simulink model "lb3"  (R2023b)
settings: Solver=ode15s  StartTime=0.0  StopTime=10.0  MaxStep=1e-5  RelTol=1e-3
values from neighbouring files (symbols this model uses):
  C = [0, 1, 0, 0]    [lw3_1.m]
  H = acker(A, B, p_reg)    [lw3_1.m]    (also in lw3_2.m = zeros(1,4))
  K = acker(A', C', poles_obs)'    [lw3_1.m]
  x0 = [1; 0; 0; 0]    [lw3_1.m]
  x00 = [0; 0; 0; 0]    [lw3_1.m]
undefined symbols (not defined in the file or in its folder): A, B, G
settings Model: Creator=kek  LastModifiedBy=kek

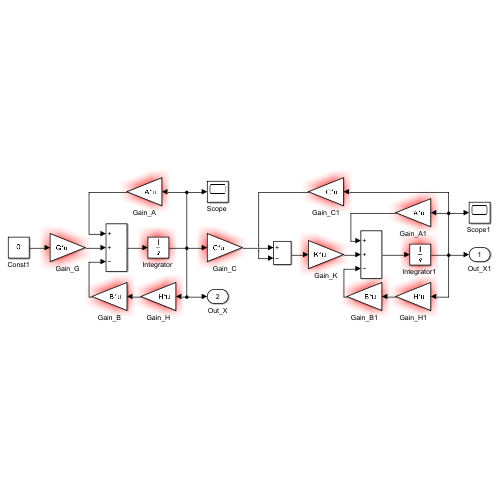
[thumbnail: Simulink's stored preview of the top-level diagram]
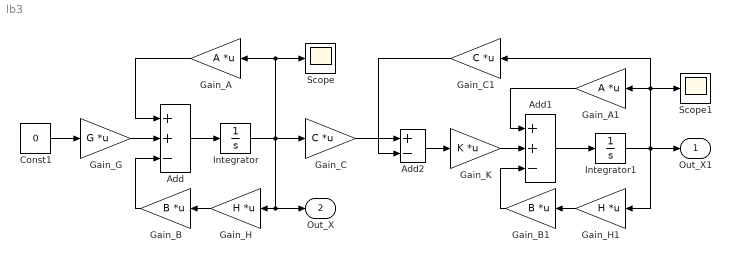
== system lb3 ==
  Add : Sum  Inputs=++-
  Add1 : Sum  Inputs=++-
  Add2 : Sum  Inputs=+-
  Const1 : Constant  Value=0
  Gain_A : Gain  Gain=A  Multiplication=Matrix(K*u)
  Gain_A1 : Gain  Gain=A  Multiplication=Matrix(K*u)
  Gain_B : Gain  Gain=B  Multiplication=Matrix(K*u)
  Gain_B1 : Gain  Gain=B  Multiplication=Matrix(K*u)
  Gain_C : Gain  Gain=C  Multiplication=Matrix(K*u)
  Gain_C1 : Gain  Gain=C  Multiplication=Matrix(K*u)
  Gain_G : Gain  Gain=G  Multiplication=Matrix(K*u)
  Gain_H : Gain  Gain=H  Multiplication=Matrix(K*u)
  Gain_H1 : Gain  Gain=H  Multiplication=Matrix(K*u)
  Gain_K : Gain  Gain=K  Multiplication=Matrix(K*u)
  "Integrator " : Integrator  InitialCondition=x0
  "Integrator1 " : Integrator  InitialCondition=x00
  "Scope " : Scope
  "Scope1 " : Scope
  Out_X1 : Outport
  Out_X : Outport  Port=2
  wires:
  "Integrator "/1 -> Gain_C/1, Out_X/1, Gain_H/1, "Scope "/1, Gain_A/1
  Add/1 -> "Integrator "/1
  Const1/1 -> Gain_G/1
  Gain_G/1 -> Add/2
  Gain_H/1 -> Gain_B/1
  Gain_A/1 -> Add/1
  Gain_B/1 -> Add/3
  Gain_H1/1 -> Gain_B1/1
  Gain_K/1 -> Add1/2
  Gain_A1/1 -> Add1/1
  Gain_B1/1 -> Add1/3
  Add1/1 -> "Integrator1 "/1
  "Integrator1 "/1 -> Out_X1/1, Gain_C1/1, "Scope1 "/1, Gain_A1/1, Gain_H1/1
  Gain_C/1 -> Add2/1
  Add2/1 -> Gain_K/1
  Gain_C1/1 -> Add2/2
